simulink model "AdaptiveCVSG"  (R2024b)
settings: Solver=ode4  StartTime=0.0  StopTime=60  FixedStep=1e-5  RelTol=1e-3
values from neighbouring files (symbols this model uses):
  mu = [6.21887134042 12.8843826697 23.6426615734 36.1444015647 49.5413580793 62.7022204476 75.4864006017 87.7683458466 99.0601107857 109.575241947 118.563685645 126.700169925 ... (200 elements, 1x200)]    [ann_model_params.mat]
  sigma = [10.4496327183 11.1148041158 11.7472409052 11.8906256492 12.3094874175 12.8461052911 13.270989651 13.5844531441 13.6128801345 13.7374243761 13.6590800387 13.618168837 ... (200 elements, 1x200)]    [ann_model_params.mat]
undefined symbols (not defined in the file or in its folder): Filter, Ls, params
libraries: neural x14, spsCurrentMeasurementLib x6, spsParallelRLCBranchLib x6, spsIGBTDiodeLib x6, spsSeriesRLCBranchLib x6, simulink x4, spsVoltageMeasurementLib x4, spsVariableInductorLib x3, spsVariableResistorLib x3, spsMeanLib x2, spsDCVoltageSourceLib x1, spsThreePhaseSourceLib x1
(part 1 of 4)
settings Model: SimulationMode=accelerator  Creator=Admin  LastModifiedBy=ACER
settings DataIOCC: SaveOutput=off  DSMLogging=off  SaveTime=off  ReturnWorkspaceOutputs=off
settings OptimizationCC: EfficientMapNaN2IntZero=off  AccelVerboseBuild=on
settings DebuggingCC: SignalInfNanChecking=error  CheckMatrixSingularityMsg=error  UnconnectedInputMsg=warning  UnconnectedOutputMsg=warning  UnconnectedLineMsg=warning
settings HardwareCC: TargetBitPerPointer=64  TargetBitPerSizeT=64  TargetBitPerPtrDiffT=64  TargetLongLongMode=on  TargetIntDivRoundTo=Zero  TargetEndianess=LittleEndian  TargetWordSize=64  TargetHWDeviceType=MATLAB Host  ProdEqTarget=off
settings ModelReferenceCC: EnableRefExpFcnMdlSchedulingChecks=on
settings SFSimCC: CustomCodeUndefinedFunction=UseInterfaceOnly
settings RTWCC: GPUComputeCapability=3.5
settings CodeAppCC: MaxIdLength=128
settings GRTTargetCC: TargetLangStandard=C89/C90 (ANSI)  CombineOutputUpdateFcns=off  GRTInterface=on

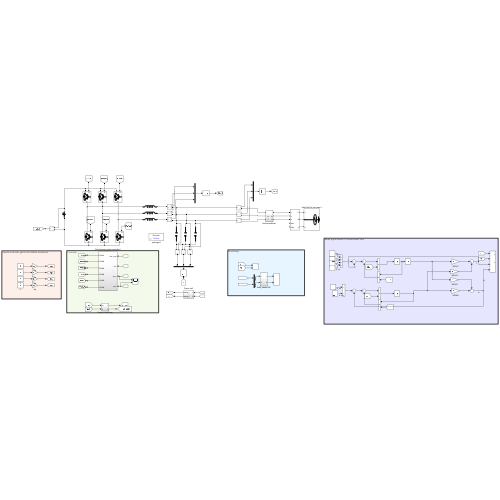
[thumbnail: Simulink's stored preview of the top-level diagram]
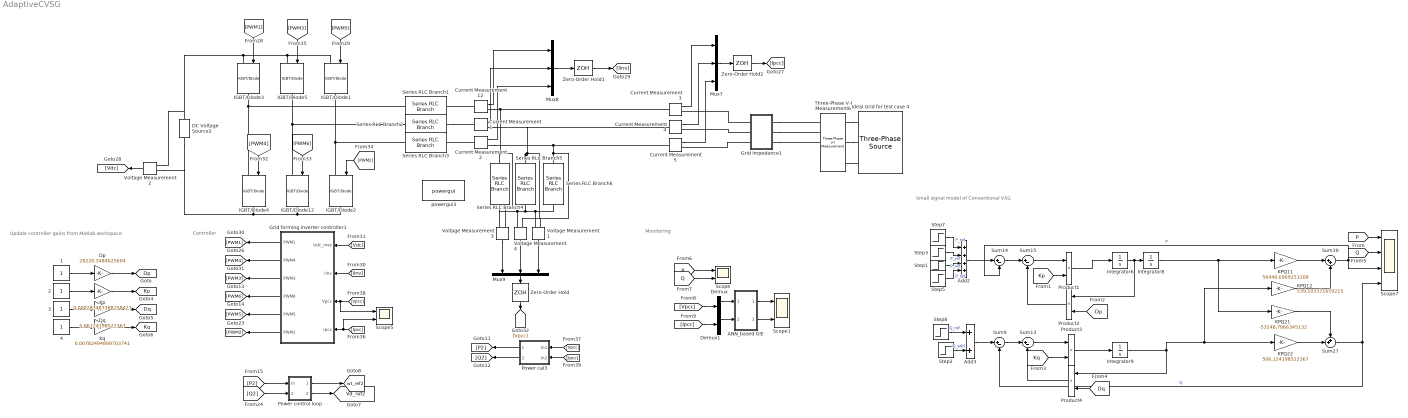
== system AdaptiveCVSG ==
  note: Update controller gains from Matlab workspace
  note: Controller
  note: Monitoring
  note: Small signal model of Conventional VSG
  {1..4} (4 alike) : Constant
  ANN_based GIE : Subsystem
  Add2 : Sum  Inputs=++++
  Add3 : Sum
  Current Measurement{1..5,12} (6 alike) : spsCurrentMeasurementLib/Current Measurement  PhasorSimulation=off  OutputType=Complex  PSBequivalent=0
  DC Voltage Source2 : spsDCVoltageSourceLib/DC Voltage Source  Amplitude=params.Vdc  Measurements=None
  Demux : Demux  Outputs=3
  Demux1 : Demux  Outputs=3
  Dp : Gain  Gain=28220.3484625604
  Dq : Gain  Gain=5.06124198522367
  Grid forming inverter controller1 : Subsystem
  Grid impedance1 : Subsystem
  IGBT/Diode{1..5,12} (6 alike) : spsIGBTDiodeLib/IGBT//Diode  Ron=1e-3  Rs=1e5  Cs=inf  Measurements=off
  Ideal Grid for test case 4 : spsThreePhaseSourceLib/Three-Phase Source  InternalConnection=Yg  VoltagePhases=off  Voltage=params.Vj*sqrt(3)  PhaseAngle=0  Voltage_phases=[25e3 25e3 25e3]/sqrt(3)  PhaseAngles_phases=[0 -120 +120]  Frequency=params.f0  NonIdealSource=off  SpecifyImpedance=on  Resistance=0.8929  Inductance=16.58e-3  ShortCircuitLevel=params.SCR*params.S_rated  BaseVoltage=params.Vll_rms  XRratio=params.XR  BusType=swing  Pref=1e3  Qref=0  Prefabc=[10e3, 10e3, 10e3]  Qrefabc=[0, 0, 0]  Qmin=-inf  Qmax=inf
  Integrator6 : Integrator
  Integrator8 : Integrator
  Integrator9 : Integrator
  KPQ11 : Gain  Gain=56440.6969251208
  KPQ12 : Gain  Gain=539.103371659215
  KPQ21 : Gain  Gain=-53248.7066345132
  KPQ22 : Gain  Gain=506.124198522367
  Kp : Gain  Gain=0.000283483388258423
  Kq : Gain  Gain=0.00782494899703741
  Mux7 : Mux  Inputs=3
  Mux8 : Mux  Inputs=3
  Mux9 : Mux  Inputs=3
  Power cal3 : Subsystem
  Power control loop : Subsystem
  Product{1..4} (4 alike) : Product
  Scope : Scope  NumInputPorts=2
  Scope1 : Scope  NumInputPorts=2
  Scope5 : Scope  NumInputPorts=2
  Scope7 : Scope  NumInputPorts=4
  Series RLC Branch1 : spsSeriesRLCBranchLib/Series RLC Branch  LConnTagsString=__new0  RConnTagsString=__new0  BranchType=L  Resistance=Filter.Rs_1  Inductance=params.Filter.Ls_1  SetiL0=off  InitialCurrent=1  Capacitance=1e-6  Setx0=off  InitialVoltage=0  Measurements=None
  Series RLC Branch2 : spsSeriesRLCBranchLib/Series RLC Branch  LConnTagsString=__new0  RConnTagsString=__new0  BranchType=L  Resistance=Filter.Rs_1  Inductance=params.Filter.Ls_1  SetiL0=off  InitialCurrent=1  Capacitance=1e-6  Setx0=off  InitialVoltage=0  Measurements=None
  Series RLC Branch3 : spsSeriesRLCBranchLib/Series RLC Branch  LConnTagsString=__new0  RConnTagsString=__new0  BranchType=L  Resistance=Filter.Rs_1  Inductance=params.Filter.Ls_1  SetiL0=off  InitialCurrent=1  Capacitance=1e-6  Setx0=off  InitialVoltage=0  Measurements=None
  Series RLC Branch4 : spsSeriesRLCBranchLib/Series RLC Branch  LConnTagsString=__new0  RConnTagsString=__new0  BranchType=C  Resistance=1  Inductance=Ls  SetiL0=off  InitialCurrent=0  Capacitance=params.Filter.Cs  Setx0=off  InitialVoltage=0  Measurements=None
  Series RLC Branch5 : spsSeriesRLCBranchLib/Series RLC Branch  LConnTagsString=__new0  RConnTagsString=__new0  BranchType=C  Resistance=1  Inductance=Ls  SetiL0=off  InitialCurrent=0  Capacitance=params.Filter.Cs  Setx0=off  InitialVoltage=0  Measurements=None
  Series RLC Branch6 : spsSeriesRLCBranchLib/Series RLC Branch  LConnTagsString=__new0  RConnTagsString=__new0  BranchType=C  Resistance=1  Inductance=Ls  SetiL0=off  InitialCurrent=0  Capacitance=params.Filter.Cs  Setx0=off  InitialVoltage=0  Measurements=None
  Step1 : Step  Time=50  After=0.5e3  SampleTime=0
  Step2 : Step  Time=25  After=0  SampleTime=0
  Step3 : Step  Time=30  After=0.5e3  SampleTime=0
  Step5 : Step  Time=70  After=0.5e3  SampleTime=0
  Step7 : Step  Time=10  Before=2e3  After=2.5e3  SampleTime=0
  Step8 : Step  Time=50  Before=params.Qref  After=params.Qref+500  SampleTime=0
  Sum{9,13..15} (4 alike) : Sum  Inputs=|+-
  Sum27 : Sum  Inputs=++|
  Sum30 : Sum  Inputs=|++
  Three-Phase V-I Measurement6 : spsThreePhaseVIMeasurementLib/Three-Phase V-I Measurement  VoltageMeasurement=phase-to-ground  SetLabelV=off  LabelV=Vabc  Vpu=off  VpuLL=off  CurrentMeasurement=yes  SetLabelI=off  LabelI=Iabc  Ipu=off  Pbase=100e6  Vbase=500e3  OutputType=Complex  PhasorSimulation=off  PSBequivalent=0
  Voltage Measurement{1..4} (4 alike) : spsVoltageMeasurementLib/Voltage Measurement  PhasorSimulation=off  OutputType=Complex  PSBequivalent=0
  Zero-Order Hold : ZeroOrderHold  SampleTime=5e-5
  Zero-Order Hold1 : ZeroOrderHold  SampleTime=5e-5
  Zero-Order Hold2 : ZeroOrderHold  SampleTime=5e-5
  powergui3 : sps_lib/powergui  Priority=1  SimulationMode=Discrete  SampleTime=params.Tsam  frequency=60  Iterations=50  frequencyindice=0  Pbase=100e6  ErrMax=1e-4  UnitsV=kV  UnitsW=MW  buscounter=0  FunctionMessages=off  echomessages=off  EnableUseOfTLC=off  CurrentSourceSwitches=off  DisableSnubberDevices=off  DisableRonSwitches=off  DisableVfSwitches=off  DisplayEquations=off  AutomaticDiscreteSolvers=on  SolverType=Tustin/Backward Euler (TBE)  Interpol=off  ExternalGateDelay=off  methode=off  Ts=100  x0status=blocks  SPID=on  SwTol=0  HookPort=off  NonlinearTolerance=0  nMaxIteration=15  ContinueOnMaxIteration=off  RestoreLinks=warning  ResistiveCurrentMeasurement=off  Frange=[0:2:500]  Ylog=off  Xlog=on  ShowGrid=off  save=off  variable=ZData  structure=0  ZoomFFT=off  StartTime=0.0  cycles=1  DisplayStyle=1  fundamental=60  FreqAxis=off  MaxFrequency=1000  frequencyindicesteady=1  RmsSteady=1  display=off
  tag scope: Dp=global, Dq=global, Kp=global, Kq=global, Vd_ref2=global, wt_ref2=global
  wires:
  1/1 -> Dp/1
  2/1 -> Kp/1
  3/1 -> Dq/1
  4/1 -> Kq/1
  Current Measurement12/1 -> Mux8/1
  Grid forming inverter controller1/3(PWM3) -> [PWM3]
  Current Measurement5/1 -> Mux7/3
  Current Measurement3/1 -> Mux7/1
  Current Measurement2/1 -> Mux8/3
  [Iinv] -> Grid forming inverter controller1/2(Iinv)
  [PWM2] -> IGBT/Diode2/1
  Voltage Measurement4/1 -> Mux9/2
  [PWM6] -> IGBT/Diode12/1
  Mux8/1 -> Zero-Order Hold1/1
  Grid forming inverter controller1/2("PWM4 ") -> [PWM4]
  Voltage Measurement2/1 -> [Vdc]
  [Vdc] -> Grid forming inverter controller1/1(Udc_mes)
  Power cal3/2(deltay2) -> [Q2]
  [PWM5] -> IGBT/Diode1/1
  [Ipcc] -> Power cal3/2(In2)
  Voltage Measurement3/1 -> Mux9/1
  Grid forming inverter controller1/6(PWM2) -> [PWM2]
  [PWM4] -> IGBT/Diode4/1
  Mux7/1 -> Zero-Order Hold2/1
  Current Measurement1/1 -> Mux8/2
  Grid forming inverter controller1/4("PWM6 ") -> [PWM6]
  Voltage Measurement1/1 -> Mux9/3
  Grid forming inverter controller1/1(PWM1) -> [PWM1]
  Power cal3/1(deltay1) -> [P2]
  Current Measurement4/1 -> Mux7/2
  Grid forming inverter controller1/5(PWM5) -> [PWM5]
  [PWM1] -> IGBT/Diode3/1
  [Ipcc] -> Scope5/2, Grid forming inverter controller1/4(Ipcc)
  [PWM3] -> IGBT/Diode5/1
  [Vpcc] -> Power cal3/1(In1)
  [Vpcc] -> Scope5/1, Grid forming inverter controller1/3(Vpcc)
  Dp/1 -> [Dp]
  Kp/1 -> [Kp]
  Dq/1 -> [Dq]
  Kq/1 -> [Kq]
  KPQ22/1 -> Sum27/2
  Integrator8/1 -> KPQ21/1, KPQ11/1
  Sum14/1 -> Sum15/1
  Sum30/1 -> Sum14/2, Scope7/3  "P"
  Product4/1 -> Sum13/2
  Sum13/1 -> Product3/1
  KPQ11/1 -> Sum30/1
  Integrator6/1 -> Product2/1, Integrator8/1
  Sum27/1 -> Scope7/4, Sum9/2  "Q"
  Product3/1 -> Integrator9/1
  Sum15/1 -> Product1/1
  Integrator9/1 -> KPQ12/1, KPQ22/1, Product4/1
  Product1/1 -> Integrator6/1
  Sum9/1 -> Sum13/1
  Step7/1 -> Add2/1  "P_ref"
  Step3/1 -> Add2/2  "P_ref"
  Step1/1 -> Add2/3  "P_ref"
  Step5/1 -> Add2/4  "P_ref"
  Add2/1 -> Sum14/1
  Step8/1 -> Add3/1  "Q_ref"
  Step2/1 -> Add3/2  "Q_add"
  Add3/1 -> Sum9/1
  [Kp] -> Product1/2
  [Dp] -> Product2/2
  Product2/1 -> Sum15/2
  [Dq] -> Product4/2
  [Kq] -> Product3/2
  [P] -> Scope7/1
  [Q] -> Scope7/2
  Zero-Order Hold/1 -> [Vpcc]
  Mux9/1 -> Zero-Order Hold/1
  Zero-Order Hold1/1 -> [Iinv]
  Zero-Order Hold2/1 -> [Ipcc]
  [Ipcc] -> Demux1/1
  [Vpcc] -> Demux/1
  [P] -> Scope/1
  [Q] -> Scope/2
  KPQ12/1 -> Sum30/2
  KPQ21/1 -> Sum27/1
  [P2] -> Power control loop/1(In)
  [Q2] -> Power control loop/2(In1)
  Power control loop/1(Out1) -> [wt_ref2]
  Power control loop/2(Out2) -> [Vd_ref2]
  Demux/1 -> ANN_based GIE/1(In1)
  Demux1/1 -> ANN_based GIE/2(In2)
  ANN_based GIE/1(Out1) -> Scope1/1
  ANN_based GIE/2(Out2) -> Scope1/2
  connections:
  IGBT/Diode5/LConn1 -- DC Voltage Source2/RConn1 -- Voltage Measurement2/LConn1 -- IGBT/Diode3/LConn1 -- IGBT/Diode1/LConn1
  Series RLC Branch5/LConn1 -- Current Measurement1/RConn1 -- Current Measurement4/LConn1 -- Voltage Measurement4/LConn1
  IGBT/Diode2/LConn1 -- IGBT/Diode1/RConn1 -- Series RLC Branch3/LConn1
  Current Measurement5/LConn1 -- Current Measurement2/RConn1 -- Series RLC Branch6/LConn1 -- Voltage Measurement1/LConn1
  IGBT/Diode12/LConn1 -- IGBT/Diode5/RConn1 -- Series RLC Branch2/LConn1
  IGBT/Diode4/RConn1 -- IGBT/Diode2/RConn1 -- IGBT/Diode12/RConn1 -- DC Voltage Source2/LConn1 -- Voltage Measurement2/LConn2
  Voltage Measurement1/LConn2 -- Series RLC Branch6/RConn1 -- Series RLC Branch5/RConn1 -- Voltage Measurement4/LConn2 -- Series RLC Branch4/RConn1 -- Voltage Measurement3/LConn2
  Voltage Measurement3/LConn1 -- Series RLC Branch4/LConn1 -- Current Measurement3/LConn1 -- Current Measurement12/RConn1
  IGBT/Diode4/LConn1 -- Series RLC Branch1/LConn1 -- IGBT/Diode3/RConn1
  Grid impedance1/LConn3 -- Current Measurement5/RConn1
  Three-Phase V-I Measurement6/LConn3 -- Ideal Grid for test case 4/RConn3
  Ideal Grid for test case 4/RConn1 -- Three-Phase V-I Measurement6/LConn1
  Grid impedance1/LConn2 -- Current Measurement4/RConn1
  Grid impedance1/RConn3 -- Three-Phase V-I Measurement6/RConn1
  Current Measurement12/LConn1 -- Series RLC Branch1/RConn1
  Grid impedance1/RConn1 -- Three-Phase V-I Measurement6/RConn3
  Current Measurement2/LConn1 -- Series RLC Branch3/RConn1
  Three-Phase V-I Measurement6/LConn2 -- Ideal Grid for test case 4/RConn2
  Series RLC Branch2/RConn1 -- Current Measurement1/LConn1
  Grid impedance1/RConn2 -- Three-Phase V-I Measurement6/RConn2
  Grid impedance1/LConn1 -- Current Measurement3/RConn1

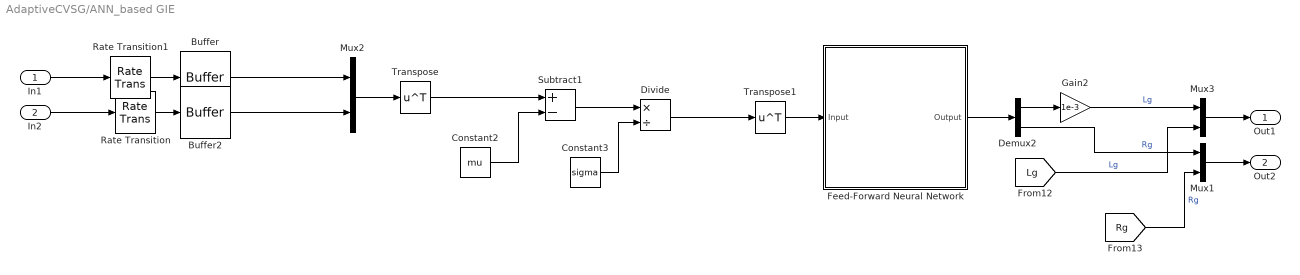
== system AdaptiveCVSG/ANN_based GIE ==
  In1 : Inport
  In2 : Inport  Port=2
  Buffer : Buffer  N=100  OutputFrames=off
  Buffer2 : Buffer  N=100  OutputFrames=off
  Constant2 : Constant  Value=mu
  Constant3 : Constant  Value=sigma
  Demux2 : Demux  Outputs=2
  Divide : Product  Inputs=*/
  Feed-Forward Neural Network : Subsystem
      mask help: Feed-Forward Neural Network
      mask Display: e = 0.06;c1 = [120 150 230]/255;c2 = ([120 150 230]+0)/383;c3 = ([120 150 230]+128)/383;patch([0 1 1 0],[0 0 1 1],c1);patch([0 1 1 1-e 1-e 0+e],[0 0 1 1-e 0+e 0+e],c2);patch([0 0 1 1-e 0+e 0+e],[0 1 1 1-e 1-e 0+e],c3);plot([0 1 1 0 0],[0 0 1 1 0]);fprintf('NNET');port_label('input',1,' Input');port_label('output',1,'Output ');
  Gain2 : Gain  Gain=1e-3
  Mux1 : Mux  Inputs=2
  Mux2 : Mux  Inputs=2
  Mux3 : Mux  Inputs=2
  Rate Transition : RateTransition  OutPortSampleTimeMultiple=20  OutPortSampleTime=2e-4
  Rate Transition1 : RateTransition  OutPortSampleTimeMultiple=20  OutPortSampleTime=2e-4
  Subtract1 : Sum  Inputs=+-
  Transpose : Math  Operator=transpose
  Transpose1 : Math  Operator=transpose
  Out1 : Outport
  Out2 : Outport  Port=2
  wires:
  Divide/1 -> Transpose1/1
  [Rg] -> Mux1/2  "Rg"
  Feed-Forward Neural Network/1(Output) -> Demux2/1
  Subtract1/1 -> Divide/1
  Transpose/1 -> Subtract1/1
  [Lg] -> Mux3/2  "Lg"
  Gain2/1 -> Mux3/1  "Lg"
  Demux2/2 -> Mux1/1  "Rg"
  Rate Transition/1 -> Buffer2/1
  Buffer2/1 -> Mux2/2
  Buffer/1 -> Mux2/1
  Constant3/1 -> Divide/2
  Transpose1/1 -> Feed-Forward Neural Network/1(Input)
  In1/1 -> Rate Transition1/1
  Constant2/1 -> Subtract1/2
  Mux2/1 -> Transpose/1
  Rate Transition1/1 -> Buffer/1
  Demux2/1 -> Gain2/1
  Mux1/1 -> Out2/1
  Mux3/1 -> Out1/1
  In2/1 -> Rate Transition/1

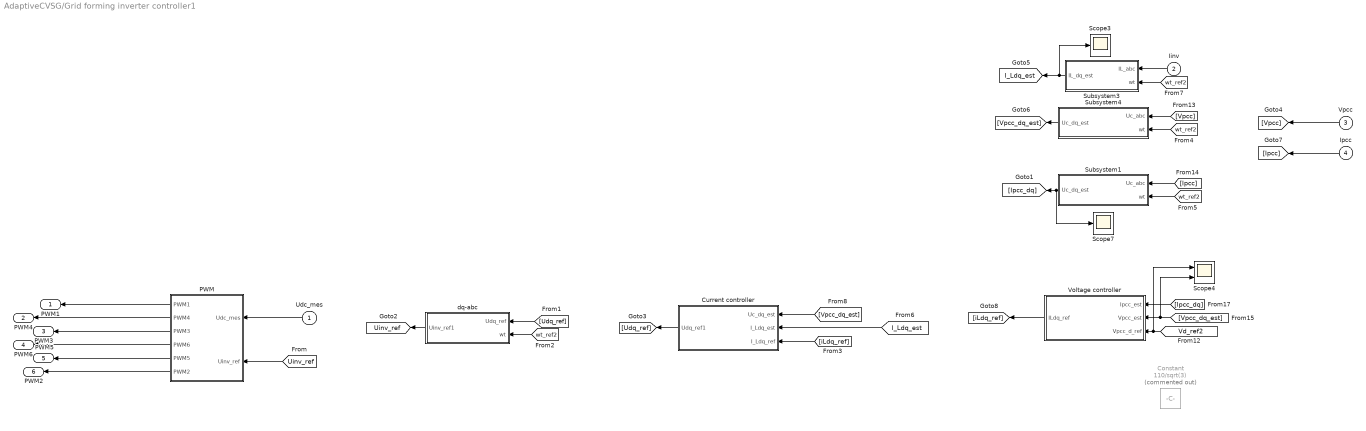
== system AdaptiveCVSG/Grid forming inverter controller1 ==
  Udc_mes : Inport
  Iinv : Inport  Port=2
  Vpcc : Inport  Port=3
  Ipcc : Inport  Port=4
  Constant : Constant  Commented=on  Value=110/sqrt(3)
  Current controller : Subsystem
  PWM : Subsystem
  Scope3 : Scope
  Scope4 : Scope  NumInputPorts=2
  Scope7 : Scope
  Subsystem1 : Subsystem
  Subsystem3 : Subsystem
  Subsystem4 : Subsystem
  Voltage controller : Subsystem
  dq-abc : Subsystem
  PWM1 : Outport
  "PWM4 " : Outport  Port=2
  PWM3 : Outport  Port=3
  "PWM6 " : Outport  Port=4
  PWM5 : Outport  Port=5
  PWM2 : Outport  Port=6
  tag scope: I_Ldq_est=global, Uinv_ref=global
  wires:
  [Vd_ref2] -> Voltage controller/3(Vpcc_d_ref), Scope4/1
  [Ipcc] -> Subsystem1/1(Uc_abc)
  [Vpcc] -> Subsystem4/1(Uc_abc)
  Ipcc/1 -> [Ipcc]
  Vpcc/1 -> [Vpcc]
  Subsystem1/1(Uc_dq_est) -> Scope7/1, [Ipcc_dq]
  [wt_ref2] -> Subsystem1/2(wt)
  [iLdq_ref] -> Current controller/3(I_Ldq_ref)
  [Vpcc_dq_est] -> Voltage controller/2(Vpcc_est), Scope4/2
  Voltage controller/1(ILdq_ref) -> [iLdq_ref]
  [Ipcc_dq] -> Voltage controller/1(Ipcc_est)
  [Uinv_ref] -> PWM/2(Uinv_ref)
  [Udq_ref] -> dq-abc/1(Udq_ref)
  PWM/2("PWM4 ") -> "PWM4 "/1
  PWM/6(PWM2) -> PWM2/1
  PWM/5(PWM5) -> PWM5/1
  PWM/1(PWM1) -> PWM1/1
  [wt_ref2] -> Subsystem4/2(wt)
  Subsystem3/1(IL_dq_est) -> [I_Ldq_est], Scope3/1
  PWM/3(PWM3) -> PWM3/1
  Iinv/1 -> Subsystem3/1(IL_abc)
  [wt_ref2] -> dq-abc/2(wt)
  dq-abc/1(Uinv_ref1) -> [Uinv_ref]
  [wt_ref2] -> Subsystem3/2(wt)
  Current controller/1(Udq_ref1) -> [Udq_ref]
  Subsystem4/1(Uc_dq_est) -> [Vpcc_dq_est]
  [I_Ldq_est] -> Current controller/2(I_Ldq_est)
  Udc_mes/1 -> PWM/1(Udc_mes)
  PWM/4("PWM6 ") -> "PWM6 "/1
  [Vpcc_dq_est] -> Current controller/1(Uc_dq_est)

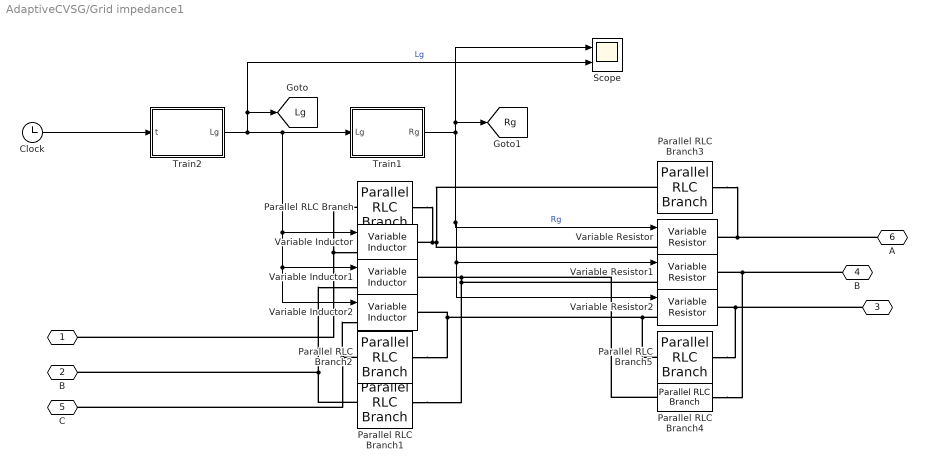
== system AdaptiveCVSG/Grid impedance1 ==
  Clock : Clock
      settings: Decimation=150
  Parallel RLC Branch{,1..5} (6 alike) : spsParallelRLCBranchLib/Parallel RLC Branch  LConnTagsString=a  RConnTagsString=__new0  BranchType=R  Resistance=1e6  Inductance=1e-3  SetiL0=off  InitialCurrent=0  Capacitance=1e-6  Setx0=off  InitialVoltage=0  Measurements=None
  Scope : Scope  NumInputPorts=2
  Train1 : MATLAB Function  TreatAsAtomicUnit=on
  Train2 : MATLAB Function  TreatAsAtomicUnit=on
  Variable Inductor : spsVariableInductorLib/Variable Inductor  methode=Backward Euler  Labsmin=1e-6  Initialize=off  iL0=0  L0=1e-3  Vl0=-0.0024759
  Variable Inductor1 : spsVariableInductorLib/Variable Inductor  methode=Backward Euler  Labsmin=1e-6  Initialize=off  iL0=0  L0=1e-3  Vl0=67.3622
  Variable Inductor2 : spsVariableInductorLib/Variable Inductor  methode=Backward Euler  Labsmin=1e-6  Initialize=off  iL0=0  L0=1e-3  Vl0=-67.3597
  Variable Resistor : spsVariableResistorLib/Variable Resistor  Rabsmin=1e-3
  Variable Resistor1 : spsVariableResistorLib/Variable Resistor  Rabsmin=1e-3
  Variable Resistor2 : spsVariableResistorLib/Variable Resistor  Rabsmin=1e-3
  "   " : PMIOPort  Side=Left
  "   B" : PMIOPort  Port=2  Side=Left
  "  " : PMIOPort  Port=3  Side=Right
  "  B" : PMIOPort  Port=4  Side=Right
  "   C" : PMIOPort  Port=5  Side=Left
  "  A" : PMIOPort  Port=6  Side=Right
  tag scope: Lg=global, Rg=global
  wires:
  Train2/1(Lg) -> Train1/1(Lg), Variable Inductor2/1, Variable Inductor1/1, Variable Inductor/1, [Lg], Scope/2  "Lg"
  Clock/1 -> Train2/1(t)
  Train1/1(Rg) -> Scope/1, [Rg], Variable Resistor2/1, Variable Resistor1/1, Variable Resistor/1  "Rg"
  connections:
  Parallel RLC Branch2/LConn1 -- "   C"/RConn1 -- Variable Inductor2/LConn1
  Parallel RLC Branch1/LConn1 -- "   B"/RConn1 -- Variable Inductor1/LConn1
  Parallel RLC Branch/RConn1 -- Variable Resistor/LConn1 -- Parallel RLC Branch3/LConn1 -- Variable Inductor/RConn1
  Parallel RLC Branch/LConn1 -- "   "/RConn1 -- Variable Inductor/LConn1
  "  A"/RConn1 -- Parallel RLC Branch3/RConn1 -- Variable Resistor/RConn1
  "  "/RConn1 -- Parallel RLC Branch5/RConn1 -- Variable Resistor2/RConn1
  "  B"/RConn1 -- Parallel RLC Branch4/RConn1 -- Variable Resistor1/RConn1
  Parallel RLC Branch2/RConn1 -- Variable Inductor2/RConn1 -- Parallel RLC Branch5/LConn1 -- Variable Resistor2/LConn1
  Parallel RLC Branch1/RConn1 -- Parallel RLC Branch4/LConn1 -- Variable Inductor1/RConn1 -- Variable Resistor1/LConn1

== system AdaptiveCVSG/Power cal3 ==
  In1 : Inport
  In2 : Inport  Port=2
  Demux10 : Demux  Outputs=3
  Demux11 : Demux  Outputs=3
  Subsystem8 : Subsystem
  Subsystem9 : Subsystem
  p3 : Subsystem
  q3 : Subsystem
  deltay1 : Outport
  deltay2 : Outport  Port=2
  wires:
  Subsystem8/1(xalpha) -> p3/3(xalpha), q3/3(xalpha)
  Demux11/3 -> Subsystem9/3(xc)
  Subsystem8/2(xbeta) -> p3/4(xbeta), q3/4(xbeta)
  Demux10/2 -> Subsystem8/2(xb)
  Subsystem9/1(xalpha) -> p3/1(Alpha), q3/1(Alpha)
  Demux10/3 -> Subsystem8/3(xc)
  p3/1(deltay1) -> deltay1/1
  Subsystem9/2(xbeta) -> p3/2(Beta), q3/2(Beta)
  Demux11/1 -> Subsystem9/1(xa)
  Demux11/2 -> Subsystem9/2(xb)
  Demux10/1 -> Subsystem8/1(xa)
  q3/1(deltay2) -> deltay2/1
  In2/1 -> Demux10/1
  In1/1 -> Demux11/1

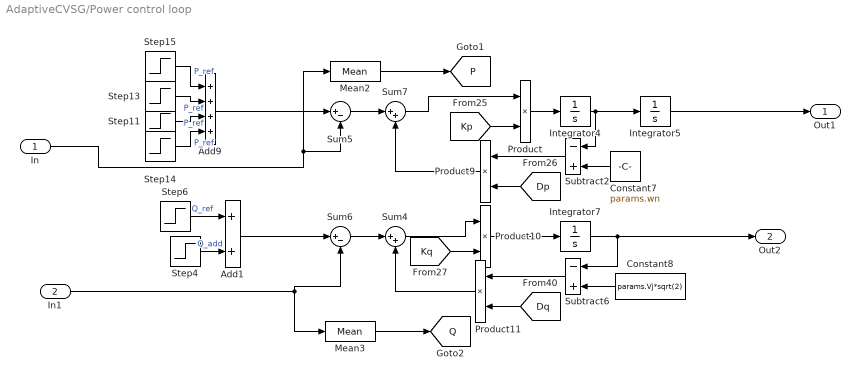
== system AdaptiveCVSG/Power control loop ==
  In : Inport
  In1 : Inport  Port=2
  Add1 : Sum
  Add9 : Sum  Inputs=++++
  Constant7 : Constant  Value=params.wn
  Constant8 : Constant  Value=params.Vj*sqrt(2)
  Integrator4 : Integrator
  Integrator5 : Integrator  InitialCondition=0.034393045493197
  Integrator7 : Integrator  InitialCondition=110.742
  Mean2 : spsMeanLib/Mean  Freq=60  Vinit=0  Ts=0
  Mean3 : spsMeanLib/Mean  Freq=60  Vinit=0  Ts=0
  Product{,9..11} (4 alike) : Product
  Step11 : Step  Time=70  After=0.5e3  SampleTime=0
  Step13 : Step  Time=30  After=0.5e3  SampleTime=0
  Step14 : Step  Time=70  After=0.5e3  SampleTime=0
  Step15 : Step  Time=10  Before=2e3  After=2.5e3  SampleTime=0
  Step4 : Step  Time=25  After=0  SampleTime=0
  Step6 : Step  Time=50  Before=params.Qref  After=params.Qref+500  SampleTime=0
  Subtract2 : Sum  Inputs=-+
  Subtract6 : Sum  Inputs=-+
  Sum4 : Sum  Inputs=|++
  Sum5 : Sum  Inputs=|+-
  Sum6 : Sum  Inputs=|+-
  Sum7 : Sum  Inputs=|++
  Out1 : Outport
  Out2 : Outport  Port=2
  tag scope: P=global, Q=global
  wires:
  [Kq] -> Product10/2
  Step13/1 -> Add9/2  "P_ref"
  In1/1 -> Sum6/2, Mean3/1
  [Kp] -> Product/2
  Product9/1 -> Sum7/2
  Step15/1 -> Add9/1  "P_ref"
  [Dp] -> Product9/2
  Subtract2/1 -> Product9/1
  Integrator7/1 -> Out2/1, Subtract6/1
  Constant7/1 -> Subtract2/2
  Sum5/1 -> Sum7/1
  Subtract6/1 -> Product11/1
  Integrator4/1 -> Integrator5/1, Subtract2/1
  Add9/1 -> Sum5/1
  Sum7/1 -> Product/1
  Add1/1 -> Sum6/1
  Product/1 -> Integrator4/1
  Step6/1 -> Add1/1  "Q_ref"
  Step11/1 -> Add9/3  "P_ref"
  Mean2/1 -> [P]
  Constant8/1 -> Subtract6/2
  Step4/1 -> Add1/2  "Q_add"
  Sum4/1 -> Product10/1
  [Dq] -> Product11/2
  Product11/1 -> Sum4/2
  Mean3/1 -> [Q]
  In/1 -> Mean2/1, Sum5/2
  Step14/1 -> Add9/4  "P_ref"
  Product10/1 -> Integrator7/1
  Sum6/1 -> Sum4/1
  Integrator5/1 -> Out1/1

== system AdaptiveCVSG/ANN_based GIE/Feed-Forward Neural Network ==
  Input : Inport  PortDimensions=200
      mask Display: e = 0.06;c1 = [120 230 180]/255;c2 = ([120 230 180]+0)/(256+128);c3 = ([120 230 180]+128)/(256+128);patch([0 1 1 0],[0 0 1 1],c1);patch([0 1 1 1-e 1-e 0+e],[0 0 1 1-e 0+e 0+e],c2);patch([0 0 1 1-e 0+e 0+e],[0 1 1 1-e 1-e 0+e],c3);plot([0 1 1 0 0],[0 0 1 1 0]);
  Layer 1 : Subsystem
      mask Display: e = 0.06;c1 = [120 150 230]/255;c2 = ([120 150 230]+0)/383;c3 = ([120 150 230]+128)/383;patch([0 1 1 0],[0 0 1 1],c1);patch([0 1 1 1-e 1-e 0+e],[0 0 1 1-e 0+e 0+e],c2);patch([0 0 1 1-e 0+e 0+e],[0 1 1 1-e 1-e 0+e],c3);plot([0 1 1 0 0],[0 0 1 1 0]);
  Layer 2 : Subsystem
      mask Display: e = 0.06;c1 = [120 150 230]/255;c2 = ([120 150 230]+0)/383;c3 = ([120 150 230]+128)/383;patch([0 1 1 0],[0 0 1 1],c1);patch([0 1 1 1-e 1-e 0+e],[0 0 1 1-e 0+e 0+e],c2);patch([0 0 1 1-e 0+e 0+e],[0 1 1 1-e 1-e 0+e],c3);plot([0 1 1 0 0],[0 0 1 1 0]);
  Process Input 1 : Subsystem
      mask Display: e = 0.06;c1 = [120 150 230]/255;c2 = ([120 150 230]+0)/383;c3 = ([120 150 230]+128)/383;patch([0 1 1 0],[0 0 1 1],c1);patch([0 1 1 1-e 1-e 0+e],[0 0 1 1-e 0+e 0+e],c2);patch([0 0 1 1-e 0+e 0+e],[0 1 1 1-e 1-e 0+e],c3);plot([0 1 1 0 0],[0 0 1 1 0]);
  Process Output 1 : Subsystem
      mask Display: e = 0.06;c1 = [120 150 230]/255;c2 = ([120 150 230]+0)/383;c3 = ([120 150 230]+128)/383;patch([0 1 1 0],[0 0 1 1],c1);patch([0 1 1 1-e 1-e 0+e],[0 0 1 1-e 0+e 0+e],c2);patch([0 0 1 1-e 0+e 0+e],[0 1 1 1-e 1-e 0+e],c3);plot([0 1 1 0 0],[0 0 1 1 0]);
  Output : Outport  InitialOutput=[0;0]
      mask Display: e = 0.06;c1 = [120 230 180]/255;c2 = ([120 230 180]+0)/(256+128);c3 = ([120 230 180]+128)/(256+128);patch([0 1 1 0],[0 0 1 1],c1);patch([0 1 1 1-e 1-e 0+e],[0 0 1 1-e 0+e 0+e],c2);patch([0 0 1 1-e 0+e 0+e],[0 1 1 1-e 1-e 0+e],c3);plot([0 1 1 0 0],[0 0 1 1 0]);
  wires:
  Input/1 -> Process Input 1/1(x)
  Process Output 1/1(y) -> Output/1
  Process Input 1/1(p) -> Layer 1/1("p{1}")
  Layer 1/1("a{1}") -> [feedback1]
  [feedback1] -> Layer 2/1("a{1} ")
  Layer 2/1("a{2}") -> Process Output 1/1(a)

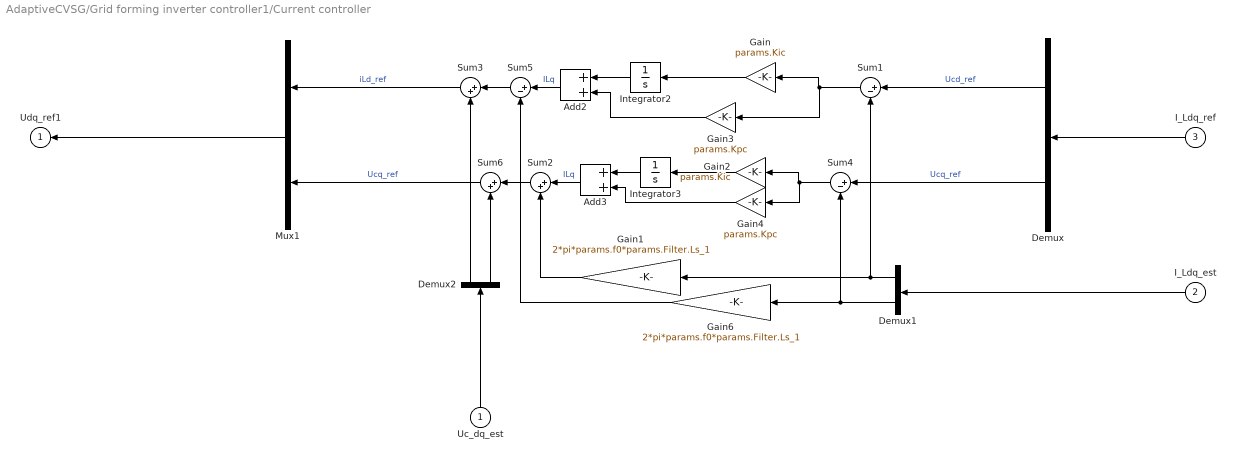
== system AdaptiveCVSG/Grid forming inverter controller1/Current controller ==
  Uc_dq_est : Inport
  I_Ldq_est : Inport  Port=2
  I_Ldq_ref : Inport  Port=3
  Add2 : Sum
  Add3 : Sum
  Demux : Demux  Outputs=2
  Demux1 : Demux  Outputs=2
  Demux2 : Demux  Outputs=2
  Gain : Gain  Gain=params.Kic
  Gain1 : Gain  Gain=2*pi*params.f0*params.Filter.Ls_1
  Gain2 : Gain  Gain=params.Kic
  Gain3 : Gain  Gain=params.Kpc
  Gain4 : Gain  Gain=params.Kpc
  Gain6 : Gain  Gain=2*pi*params.f0*params.Filter.Ls_1
  Integrator2 : Integrator
  Integrator3 : Integrator
  Mux1 : Mux  Inputs=2
  Sum1 : Sum  Inputs=|+-
  Sum2 : Sum  Inputs=|++
  Sum3 : Sum  Inputs=|++
  Sum4 : Sum  Inputs=|+-
  Sum5 : Sum  Inputs=|+-
  Sum6 : Sum  Inputs=|++
  Udq_ref1 : Outport  InitialOutput=0  VectorParamsAs1DForOutWhenUnconnected=off
  wires:
  Gain4/1 -> Add3/2
  Gain3/1 -> Add2/2
  Sum4/1 -> Gain2/1, Gain4/1
  Gain2/1 -> Integrator3/1
  Sum1/1 -> Gain/1, Gain3/1
  Gain/1 -> Integrator2/1
  Integrator3/1 -> Add3/1
  Integrator2/1 -> Add2/1
  Add3/1 -> Sum2/1  "ILq"
  Add2/1 -> Sum5/1  "ILq"
  Demux1/1 -> Gain1/1, Sum1/2
  Demux/1 -> Sum1/1  "Ucd_ref"
  Demux1/2 -> Sum4/2, Gain6/1
  Uc_dq_est/1 -> Demux2/1
  Gain6/1 -> Sum5/2
  Mux1/1 -> Udq_ref1/1
  Sum5/1 -> Sum3/1
  Demux2/1 -> Sum3/2
  Sum6/1 -> Mux1/2  "Ucq_ref"
  Gain1/1 -> Sum2/2
  Demux/2 -> Sum4/1  "Ucq_ref"
  Sum3/1 -> Mux1/1  "iLd_ref"
  I_Ldq_est/1 -> Demux1/1
  Sum2/1 -> Sum6/1
  Demux2/2 -> Sum6/2
  I_Ldq_ref/1 -> Demux/1

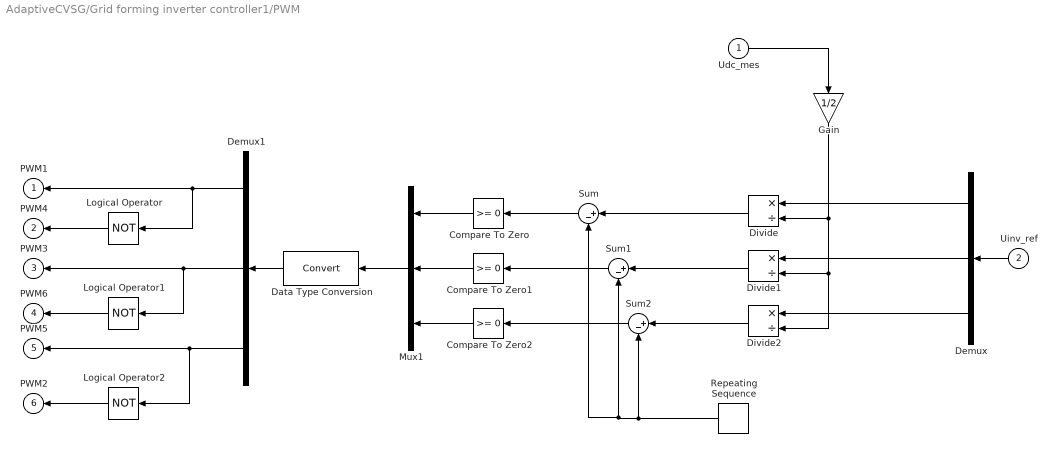
== system AdaptiveCVSG/Grid forming inverter controller1/PWM ==
  Udc_mes : Inport
  Uinv_ref : Inport  Port=2
  Compare To Zero : simulink/Logic and Bit Operations/Compare To Zero  relop=>=  OutDataTypeStr=boolean
  Compare To Zero1 : simulink/Logic and Bit Operations/Compare To Zero  relop=>=  OutDataTypeStr=boolean
  Compare To Zero2 : simulink/Logic and Bit Operations/Compare To Zero  relop=>=  OutDataTypeStr=boolean
  Data Type Conversion : DataTypeConversion  SaturateOnIntegerOverflow=off  RndMeth=Floor
  Demux : Demux  Outputs=3
  Demux1 : Demux  Outputs=3
  Divide : Product  Inputs=*/
  Divide1 : Product  Inputs=*/
  Divide2 : Product  Inputs=*/
  Gain : Gain  Gain=1/2
  Logical Operator : Logic  Operator=NOT  AllPortsSameDT=off  OutDataTypeStr=boolean
  Logical Operator1 : Logic  Operator=NOT  AllPortsSameDT=off  OutDataTypeStr=boolean
  Logical Operator2 : Logic  Operator=NOT  AllPortsSameDT=off  OutDataTypeStr=boolean
  Mux1 : Mux  Inputs=3
  Repeating Sequence : simulink/Sources/Repeating Sequence  rep_seq_t=[0 params.Ts/2 params.Ts]  rep_seq_y=[-1 1 -1]
  Sum : Sum  Inputs=|+-
  Sum1 : Sum  Inputs=|+-
  Sum2 : Sum  Inputs=|+-
  PWM1 : Outport  InitialOutput=0  VectorParamsAs1DForOutWhenUnconnected=off
  "PWM4 " : Outport  Port=2  InitialOutput=0  VectorParamsAs1DForOutWhenUnconnected=off
  PWM3 : Outport  Port=3  InitialOutput=0  VectorParamsAs1DForOutWhenUnconnected=off
  "PWM6 " : Outport  Port=4  InitialOutput=0  VectorParamsAs1DForOutWhenUnconnected=off
  PWM5 : Outport  Port=5  InitialOutput=0  VectorParamsAs1DForOutWhenUnconnected=off
  PWM2 : Outport  Port=6  InitialOutput=0  VectorParamsAs1DForOutWhenUnconnected=off
  wires:
  Compare To Zero/1 -> Mux1/1
  Data Type Conversion/1 -> Demux1/1
  Demux1/1 -> Logical Operator/1, PWM1/1
  Gain/1 -> Divide2/2, Divide1/2, Divide/2
  Sum/1 -> Compare To Zero/1
  Demux/3 -> Divide2/1
  Udc_mes/1 -> Gain/1
  Logical Operator1/1 -> "PWM6 "/1
  Logical Operator2/1 -> PWM2/1
  Demux/2 -> Divide1/1
  Compare To Zero1/1 -> Mux1/2
  Compare To Zero2/1 -> Mux1/3
  Demux1/3 -> Logical Operator2/1, PWM5/1
  Demux1/2 -> Logical Operator1/1, PWM3/1
  Uinv_ref/1 -> Demux/1
  Demux/1 -> Divide/1
  Divide1/1 -> Sum1/1
  Sum2/1 -> Compare To Zero2/1
  Logical Operator/1 -> "PWM4 "/1
  Divide/1 -> Sum/1
  Divide2/1 -> Sum2/1
  Mux1/1 -> Data Type Conversion/1
  Sum1/1 -> Compare To Zero1/1
  Repeating Sequence/1 -> Sum2/2, Sum1/2, Sum/2

== system AdaptiveCVSG/Grid forming inverter controller1/Subsystem1 ==
  Uc_abc : Inport
  wt : Inport  Port=2
  Demux : Demux  Outputs=3
  Mux1 : Mux  Inputs=2
  Subsystem1 : Subsystem
  Subsystem2 : Subsystem
  Uc_dq_est : Outport  InitialOutput=0  VectorParamsAs1DForOutWhenUnconnected=off
  wires:
  Subsystem2/2(xq) -> Mux1/2
  Demux/2 -> Subsystem1/2(xb)
  Subsystem1/1(xalpha) -> Subsystem2/1(xalpha)
  Uc_abc/1 -> Demux/1
  Demux/1 -> Subsystem1/1(xa)
  Subsystem1/2(xbeta) -> Subsystem2/2(xbeta)
  Subsystem2/1(xd) -> Mux1/1
  Demux/3 -> Subsystem1/3(xc)
  wt/1 -> Subsystem2/3(wt)
  Mux1/1 -> Uc_dq_est/1

== system AdaptiveCVSG/Grid forming inverter controller1/Subsystem3 ==
  IL_abc : Inport
  wt : Inport  Port=2
  Demux : Demux  Outputs=3
  Mux1 : Mux  Inputs=2
  Subsystem1 : Subsystem
  Subsystem2 : Subsystem
  IL_dq_est : Outport  InitialOutput=0  VectorParamsAs1DForOutWhenUnconnected=off
  wires:
  Subsystem2/1(xd) -> Mux1/1
  Subsystem2/2(xq) -> Mux1/2
  Subsystem1/1(xalpha) -> Subsystem2/1(xalpha)
  Demux/2 -> Subsystem1/2(xb)
  Mux1/1 -> IL_dq_est/1
  Subsystem1/2(xbeta) -> Subsystem2/2(xbeta)
  Demux/1 -> Subsystem1/1(xa)
  wt/1 -> Subsystem2/3(wt)
  IL_abc/1 -> Demux/1
  Demux/3 -> Subsystem1/3(xc)

== system AdaptiveCVSG/Grid forming inverter controller1/Subsystem4 ==
  Uc_abc : Inport
  wt : Inport  Port=2
  Demux : Demux  Outputs=3
  Mux1 : Mux  Inputs=2
  Subsystem1 : Subsystem
  Subsystem2 : Subsystem
  Uc_dq_est : Outport  InitialOutput=0  VectorParamsAs1DForOutWhenUnconnected=off
  wires:
  Mux1/1 -> Uc_dq_est/1
  wt/1 -> Subsystem2/3(wt)
  Demux/3 -> Subsystem1/3(xc)
  Subsystem2/1(xd) -> Mux1/1
  Subsystem1/2(xbeta) -> Subsystem2/2(xbeta)
  Demux/1 -> Subsystem1/1(xa)
  Uc_abc/1 -> Demux/1
  Subsystem1/1(xalpha) -> Subsystem2/1(xalpha)
  Demux/2 -> Subsystem1/2(xb)
  Subsystem2/2(xq) -> Mux1/2

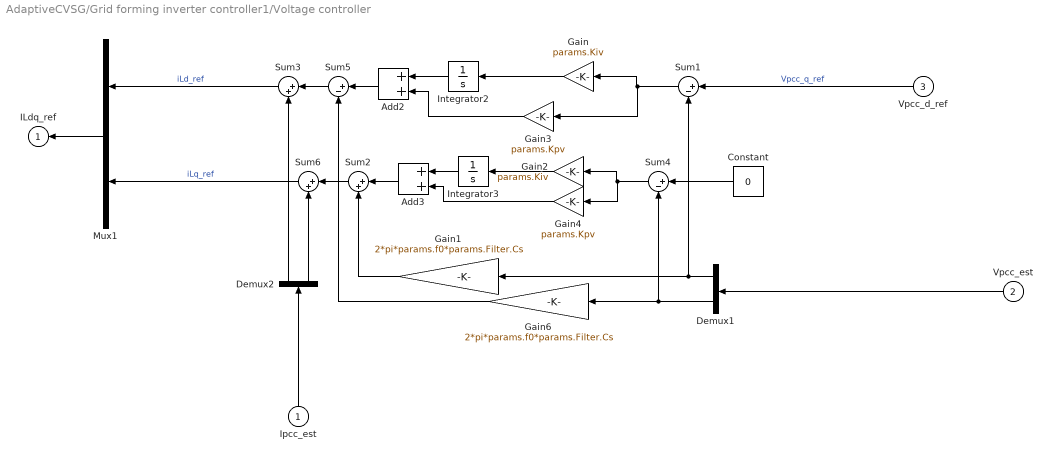
== system AdaptiveCVSG/Grid forming inverter controller1/Voltage controller ==
  Ipcc_est : Inport
  Vpcc_est : Inport  Port=2
  Vpcc_d_ref : Inport  Port=3
  Add2 : Sum
  Add3 : Sum
  Constant : Constant  Value=0
  Demux1 : Demux  Outputs=2
  Demux2 : Demux  Outputs=2
  Gain : Gain  Gain=params.Kiv
  Gain1 : Gain  Gain=2*pi*params.f0*params.Filter.Cs
  Gain2 : Gain  Gain=params.Kiv
  Gain3 : Gain  Gain=params.Kpv
  Gain4 : Gain  Gain=params.Kpv
  Gain6 : Gain  Gain=2*pi*params.f0*params.Filter.Cs
  Integrator2 : Integrator
  Integrator3 : Integrator
  Mux1 : Mux  Inputs=2
  Sum1 : Sum  Inputs=|+-
  Sum2 : Sum  Inputs=|++
  Sum3 : Sum  Inputs=|++
  Sum4 : Sum  Inputs=|+-
  Sum5 : Sum  Inputs=|+-
  Sum6 : Sum  Inputs=|++
  ILdq_ref : Outport  InitialOutput=0  VectorParamsAs1DForOutWhenUnconnected=off
  wires:
  Constant/1 -> Sum4/1
  Vpcc_d_ref/1 -> Sum1/1  "Vpcc_q_ref"
  Demux2/2 -> Sum6/2
  Sum2/1 -> Sum6/1
  Vpcc_est/1 -> Demux1/1
  Sum3/1 -> Mux1/1  "iLd_ref"
  Gain1/1 -> Sum2/2
  Sum6/1 -> Mux1/2  "iLq_ref"
  Demux2/1 -> Sum3/2
  Sum5/1 -> Sum3/1
  Mux1/1 -> ILdq_ref/1
  Gain6/1 -> Sum5/2
  Ipcc_est/1 -> Demux2/1
  Demux1/2 -> Gain6/1, Sum4/2
  Demux1/1 -> Sum1/2, Gain1/1
  Add2/1 -> Sum5/1
  Add3/1 -> Sum2/1
  Integrator2/1 -> Add2/1
  Integrator3/1 -> Add3/1
  Gain/1 -> Integrator2/1
  Sum1/1 -> Gain3/1, Gain/1
  Gain2/1 -> Integrator3/1
  Sum4/1 -> Gain4/1, Gain2/1
  Gain3/1 -> Add2/2
  Gain4/1 -> Add3/2

== system AdaptiveCVSG/Grid forming inverter controller1/dq-abc ==
  Udq_ref : Inport
  wt : Inport  Port=2
  Subsystem2 : Subsystem
  Subsystem3 : Subsystem
  Uinv_ref1 : Outport  InitialOutput=0  VectorParamsAs1DForOutWhenUnconnected=off
  wires:
  Udq_ref/1 -> Subsystem2/1(xdq)
  Subsystem3/1(xabc) -> Uinv_ref1/1
  Subsystem2/1(xalbe) -> Subsystem3/1(xalbe)
  wt/1 -> Subsystem2/2(wt)

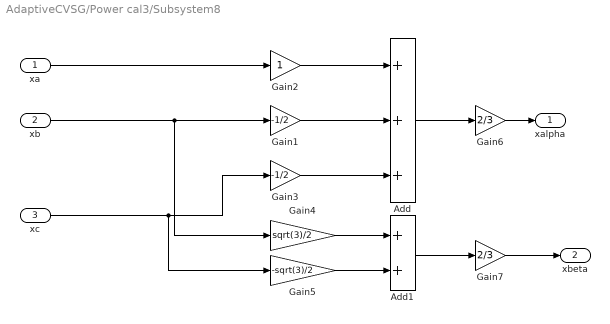
== system AdaptiveCVSG/Power cal3/Subsystem8 ==
  xa : Inport
  xb : Inport  Port=2
  xc : Inport  Port=3
  Add : Sum  Inputs=+++
  Add1 : Sum
  Gain1 : Gain  Gain=-1/2
  Gain2 : Gain
  Gain3 : Gain  Gain=-1/2
  Gain4 : Gain  Gain=sqrt(3)/2
  Gain5 : Gain  Gain=-sqrt(3)/2
  Gain6 : Gain  Gain=2/3
  Gain7 : Gain  Gain=2/3
  xalpha : Outport  VectorParamsAs1DForOutWhenUnconnected=off
  xbeta : Outport  Port=2  VectorParamsAs1DForOutWhenUnconnected=off
  wires:
  xa/1 -> Gain2/1
  Gain7/1 -> xbeta/1
  Gain4/1 -> Add1/1
  Add/1 -> Gain6/1
  Gain2/1 -> Add/1
  Gain5/1 -> Add1/2
  xb/1 -> Gain1/1, Gain4/1
  Gain1/1 -> Add/2
  Gain3/1 -> Add/3
  Add1/1 -> Gain7/1
  Gain6/1 -> xalpha/1
  xc/1 -> Gain3/1, Gain5/1

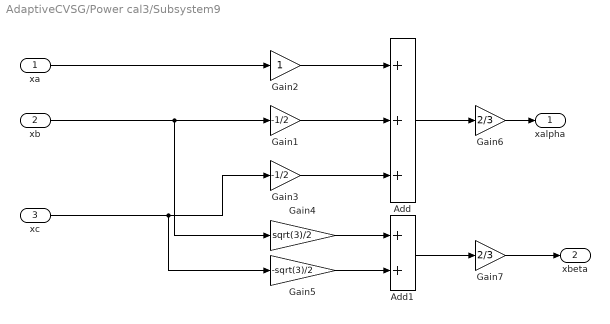
== system AdaptiveCVSG/Power cal3/Subsystem9 ==
  xa : Inport
  xb : Inport  Port=2
  xc : Inport  Port=3
  Add : Sum  Inputs=+++
  Add1 : Sum
  Gain1 : Gain  Gain=-1/2
  Gain2 : Gain
  Gain3 : Gain  Gain=-1/2
  Gain4 : Gain  Gain=sqrt(3)/2
  Gain5 : Gain  Gain=-sqrt(3)/2
  Gain6 : Gain  Gain=2/3
  Gain7 : Gain  Gain=2/3
  xalpha : Outport  VectorParamsAs1DForOutWhenUnconnected=off
  xbeta : Outport  Port=2  VectorParamsAs1DForOutWhenUnconnected=off
  wires:
  xc/1 -> Gain5/1, Gain3/1
  Gain6/1 -> xalpha/1
  Add1/1 -> Gain7/1
  Gain3/1 -> Add/3
  Gain1/1 -> Add/2
  xb/1 -> Gain4/1, Gain1/1
  Gain5/1 -> Add1/2
  Gain2/1 -> Add/1
  Add/1 -> Gain6/1
  Gain4/1 -> Add1/1
  Gain7/1 -> xbeta/1
  xa/1 -> Gain2/1

== system AdaptiveCVSG/Power cal3/p3 ==
  Alpha : Inport
  Beta : Inport  Port=2
  xalpha : Inport  Port=3
  xbeta : Inport  Port=4
  Add : Sum
  Gain : Gain  Gain=3/2
  Product : Product
  Product1 : Product
  deltay1 : Outport
  wires:
  xbeta/1 -> Product1/2
  Beta/1 -> Product1/1
  xalpha/1 -> Product/2
  Alpha/1 -> Product/1
  Add/1 -> Gain/1
  Product/1 -> Add/1
  Gain/1 -> deltay1/1
  Product1/1 -> Add/2

== system AdaptiveCVSG/Power cal3/q3 ==
  Alpha : Inport
  Beta : Inport  Port=2
  xalpha : Inport  Port=3
  xbeta : Inport  Port=4
  Add : Sum  Inputs=+-
  Gain : Gain  Gain=3/2
  Product : Product
  Product1 : Product
  deltay2 : Outport
  wires:
  xbeta/1 -> Product1/2
  Alpha/1 -> Product1/1
  xalpha/1 -> Product/2
  Beta/1 -> Product/1
  Product1/1 -> Add/2
  Gain/1 -> deltay2/1
  Product/1 -> Add/1
  Add/1 -> Gain/1

== system AdaptiveCVSG/ANN_based GIE/Feed-Forward Neural Network/Layer 1 ==
  "p{1}" : Inport  PortDimensions=200
      mask Display: e = 0.06;c1 = [120 230 180]/255;c2 = ([120 230 180]+0)/(256+128);c3 = ([120 230 180]+128)/(256+128);patch([0 1 1 0],[0 0 1 1],c1);patch([0 1 1 1-e 1-e 0+e],[0 0 1 1-e 0+e 0+e],c2);patch([0 0 1 1-e 0+e 0+e],[0 1 1 1-e 1-e 0+e],c3);plot([0 1 1 0 0],[0 0 1 1 0]);
  Delays 1 : Subsystem
      mask Display: e = 0.06;c1 = [120 150 230]/255;c2 = ([120 150 230]+0)/383;c3 = ([120 150 230]+128)/383;patch([0 1 1 0],[0 0 1 1],c1);patch([0 1 1 1-e 1-e 0+e],[0 0 1 1-e 0+e 0+e],c2);patch([0 0 1 1-e 0+e 0+e],[0 1 1 1-e 1-e 0+e],c3);plot([0 1 1 0 0],[0 0 1 1 0]);disp('0');
  "IW{1,1}" : Subsystem
      mask Display: e = 0.06;c1 = [120 150 230]/255;c2 = ([120 150 230]+0)/383;c3 = ([120 150 230]+128)/383;patch([0 1 1 0],[0 0 1 1],c1);patch([0 1 1 1-e 1-e 0+e],[0 0 1 1-e 0+e 0+e],c2);patch([0 0 1 1-e 0+e 0+e],[0 1 1 1-e 1-e 0+e],c3);plot([0 1 1 0 0],[0 0 1 1 0]);disp('W');
  "b{1}" : Constant  Value=[-0.00534233011079685883581991134860800229944288730621337890625;0.6074929940111370996191908488981425762176513671875;0.0710144594284652652671496753100655041635036468505859375;0.043061977666802607467300134658216848038136959075927734375;0.06509617719122302859080519965573330409824848175048828125;0.10239151455412874580641613420084468089044094085693359375;0.03283089443540583574066005212443997152149677276611328125;-0.117750536619440737684527675810386426746845245361328125]
      mask Display: e = 0.06;c1 = [120 150 230]/255;c2 = ([120 150 230]+0)/383;c3 = ([120 150 230]+128)/383;patch([0 1 1 0],[0 0 1 1],c1);patch([0 1 1 1-e 1-e 0+e],[0 0 1 1-e 0+e 0+e],c2);patch([0 0 1 1-e 0+e 0+e],[0 1 1 1-e 1-e 0+e],c3);plot([0 1 1 0 0],[0 0 1 1 0]);disp('b');
  netsum : Sum  Inputs=2  InputSameDT=on  SaturateOnIntegerOverflow=on  OutDataTypeStr=Inherit: Same as first input
      mask Display: e = 0.06;c1 = [120 150 230]/255;c2 = ([120 150 230]+0)/383;c3 = ([120 150 230]+128)/383;patch([0 1 1 0],[0 0 1 1],c1);patch([0 1 1 1-e 1-e 0+e],[0 0 1 1-e 0+e 0+e],c2);patch([0 0 1 1-e 0+e 0+e],[0 1 1 1-e 1-e 0+e],c3);plot([0 1 1 0 0],[0 0 1 1 0]);disp('+');
  tansig : neural/Transfer Functions/tansig
  "a{1}" : Outport  InitialOutput=[0;0;0;0;0;0;0;0]
      mask Display: e = 0.06;c1 = [120 230 180]/255;c2 = ([120 230 180]+0)/(256+128);c3 = ([120 230 180]+128)/(256+128);patch([0 1 1 0],[0 0 1 1],c1);patch([0 1 1 1-e 1-e 0+e],[0 0 1 1-e 0+e 0+e],c2);patch([0 0 1 1-e 0+e 0+e],[0 1 1 1-e 1-e 0+e],c3);plot([0 1 1 0 0],[0 0 1 1 0]);
  wires:
  "p{1}"/1 -> Delays 1/1("p{1}")
  Delays 1/1("pd{1,1}") -> "IW{1,1}"/1("pd{1,1}")
  "IW{1,1}"/1("iz{1,1}") -> netsum/1
  "b{1}"/1 -> netsum/2
  netsum/1 -> tansig/1
  tansig/1 -> "a{1}"/1

== system AdaptiveCVSG/ANN_based GIE/Feed-Forward Neural Network/Layer 2 ==
  "a{1} " : Inport  PortDimensions=8
      mask Display: e = 0.06;c1 = [120 230 180]/255;c2 = ([120 230 180]+0)/(256+128);c3 = ([120 230 180]+128)/(256+128);patch([0 1 1 0],[0 0 1 1],c1);patch([0 1 1 1-e 1-e 0+e],[0 0 1 1-e 0+e 0+e],c2);patch([0 0 1 1-e 0+e 0+e],[0 1 1 1-e 1-e 0+e],c3);plot([0 1 1 0 0],[0 0 1 1 0]);
  Delays 1 : Subsystem
      mask Display: e = 0.06;c1 = [120 150 230]/255;c2 = ([120 150 230]+0)/383;c3 = ([120 150 230]+128)/383;patch([0 1 1 0],[0 0 1 1],c1);patch([0 1 1 1-e 1-e 0+e],[0 0 1 1-e 0+e 0+e],c2);patch([0 0 1 1-e 0+e 0+e],[0 1 1 1-e 1-e 0+e],c3);plot([0 1 1 0 0],[0 0 1 1 0]);disp('0');
  "LW{2,1}" : Subsystem
      mask Display: e = 0.06;c1 = [120 150 230]/255;c2 = ([120 150 230]+0)/383;c3 = ([120 150 230]+128)/383;patch([0 1 1 0],[0 0 1 1],c1);patch([0 1 1 1-e 1-e 0+e],[0 0 1 1-e 0+e 0+e],c2);patch([0 0 1 1-e 0+e 0+e],[0 1 1 1-e 1-e 0+e],c3);plot([0 1 1 0 0],[0 0 1 1 0]);disp('W');
  "b{2}" : Constant  Value=[0.321877407050287944745292634252109564840793609619140625;0.323047937333066637055623004926019348204135894775390625]
      mask Display: e = 0.06;c1 = [120 150 230]/255;c2 = ([120 150 230]+0)/383;c3 = ([120 150 230]+128)/383;patch([0 1 1 0],[0 0 1 1],c1);patch([0 1 1 1-e 1-e 0+e],[0 0 1 1-e 0+e 0+e],c2);patch([0 0 1 1-e 0+e 0+e],[0 1 1 1-e 1-e 0+e],c3);plot([0 1 1 0 0],[0 0 1 1 0]);disp('b');
  netsum : Sum  Inputs=2  InputSameDT=on  SaturateOnIntegerOverflow=on  OutDataTypeStr=Inherit: Same as first input
      mask Display: e = 0.06;c1 = [120 150 230]/255;c2 = ([120 150 230]+0)/383;c3 = ([120 150 230]+128)/383;patch([0 1 1 0],[0 0 1 1],c1);patch([0 1 1 1-e 1-e 0+e],[0 0 1 1-e 0+e 0+e],c2);patch([0 0 1 1-e 0+e 0+e],[0 1 1 1-e 1-e 0+e],c3);plot([0 1 1 0 0],[0 0 1 1 0]);disp('+');
  purelin : neural/Transfer Functions/purelin
  "a{2}" : Outport  InitialOutput=[0;0]
      mask Display: e = 0.06;c1 = [120 230 180]/255;c2 = ([120 230 180]+0)/(256+128);c3 = ([120 230 180]+128)/(256+128);patch([0 1 1 0],[0 0 1 1],c1);patch([0 1 1 1-e 1-e 0+e],[0 0 1 1-e 0+e 0+e],c2);patch([0 0 1 1-e 0+e 0+e],[0 1 1 1-e 1-e 0+e],c3);plot([0 1 1 0 0],[0 0 1 1 0]);
  wires:
  "a{1} "/1 -> Delays 1/1("p{2}")
  Delays 1/1("pd{2,1}") -> "LW{2,1}"/1("ad{2,1}")
  "LW{2,1}"/1("lz{2,1}") -> netsum/1
  "b{2}"/1 -> netsum/2
  netsum/1 -> purelin/1
  purelin/1 -> "a{2}"/1
